simulink model "VB_RIFKF_GNSS_INS25"  (R2023a)
settings: Solver=FixedStepAuto  StartTime=0  StopTime=500  FixedStep=0.01  RelTol=1e-3
InitFcn:
  | resilient_initNavigation1216;
  | init_param;
undefined symbols (not defined in the file or in its folder): dt, g0, gam0_rad, ISUS_flag, magnitude, p, P0, P0_RIEKF, param, pd0, pe0, phi0_rad, pn0, psi, psi0_rad, state_dim, vd0, ve0, vn0
libraries: simulink_extras x68, dspstat3 x54, sharedtransform x47, simulink x43, matrix_library x9, sharedTrackingLibrary x5, dspfactors x4, aerolibconvert2 x3, aerolibtransform2 x3
(part 4 of 22)

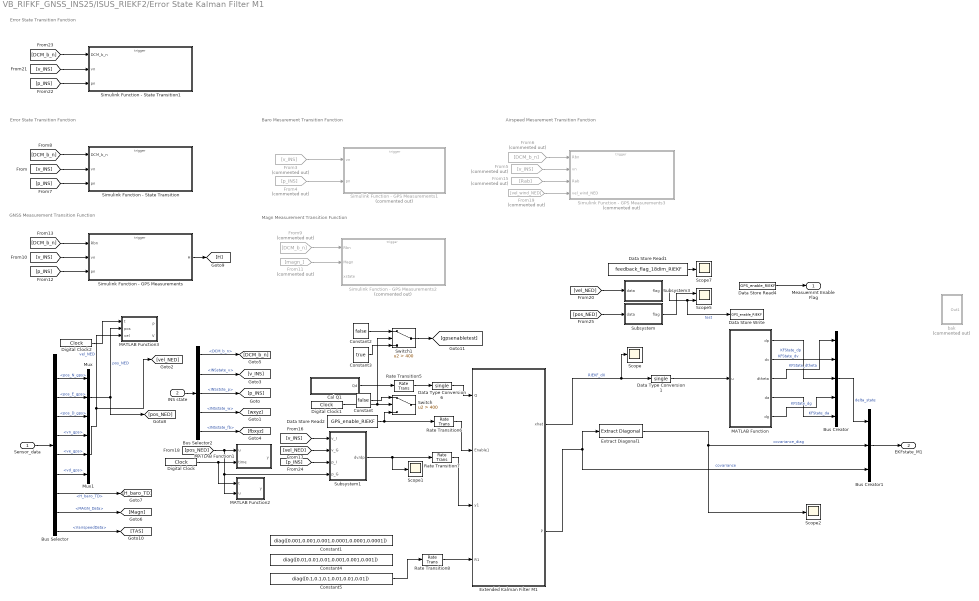
== system VB_RIFKF_GNSS_INS25/ISUS_RIEKF2/Error State Kalman Filter M1 ==
  note: Error State Transition Function
  note: GNSS Measurement Transition Function
  note: Baro Mesurement Transition Function
  note: Magn Measurement Transition Function
  note: Airspeed Mesurement Transition Function
  note: Error State Transition Function
  Sensor_data : Inport
  INS state : Inport  Port=2
  Bus Creator : BusCreator  Inputs=5
  Bus Creator1 : BusCreator  Inputs=3
  Bus Selector : BusSelector  OutputSignals=QGC_sensor_reinit,GPS_Data.pos_N_gps,GPS_Data.pos_E_gps,GPS_Data.pos_D_gps,GPS_Data.vn_gps,GPS_Data.ve_gps,GPS_Data.vd_gps,BARO_Data.H_baro_TD,MAGN_Data,VairspeedData
  Bus Selector2 : BusSelector  OutputSignals=RotationData.DCM_b_n,INSstate_v,INSstste_p,INSstate_w,INSstate_fb
  Cal Q1 : Subsystem
  Constant : Constant  Value=false
  Constant1 : Constant  Value=diag([0.001,0.001,0.001,0.0001,0.0001,0.0001])  OutDataTypeStr=single
  Constant2 : Constant  Value=false
  Constant3 : Constant  Value=true
  Constant4 : Constant  Value=diag([0.01,0.01,0.01,0.001,0.001,0.001])  OutDataTypeStr=single
  Constant5 : Constant  Value=diag([0.1,0.1,0.1,0.01,0.01,0.01])  OutDataTypeStr=single
  Data Store Read1 : DataStoreRead  DataStoreName=feedback_flag_18dim_RIEKF  IndexOptions=Index vector (dialog)  Indices=1  OutputSizes=1
  Data Store Read2 : DataStoreRead  DataStoreName=GPS_enable_RIEKF  IndexOptions=Index vector (dialog)  Indices=1  OutputSizes=1
  Data Store Read4 : DataStoreRead  DataStoreName=GPS_enable_RIEKF  IndexOptions=Index vector (dialog)  Indices=1  OutputSizes=1
  Data Store Write : DataStoreWrite  DataStoreName=GPS_enable_RIEKF  IndexOptions=Index vector (dialog)  Indices=1  OutputSizes=1
  Data Type Conversion1 : DataTypeConversion  OutDataTypeStr=single  SaturateOnIntegerOverflow=off  RndMeth=Floor
  Data Type Conversion6 : DataTypeConversion  OutDataTypeStr=single  SaturateOnIntegerOverflow=off  RndMeth=Floor
  Digital Clock : DigitalClock  SampleTime=0.01
  Digital Clock1 : DigitalClock  SampleTime=0.01
  Digital Clock2 : DigitalClock  SampleTime=0.01
  Extended Kalman Filter M1 : Subsystem  mask(Extended Kalman Filter){StateTransitionFcn=stateTransitionFcn_RIEKF, HasStateTransitionJacobianFcn=on, StateTransitionJacobianFcn=stateFcn_RIEKFJacobian, HasAdditiveProcessNoise=Nonadditive, ProcessNoise=1, HasTimeVaryingProcessNoise=on, HasStateTransitionFcnExtraArgument=0, InitialState=zeros(state_dim,1), InitialStateCovariance=P0_RIEKF, MeasurementFcn1=GPSMeasurementFcn_RIEKF, HasMeasurementJacobianFcn1=off, MeasurementJacobianFcn1=, HasMeasurementEnablePort1=on, HasAdditiveMeasurementNoise1=Nonadditive, MeasurementNoise1=1, HasTimeVaryingMeasurementNoise1=on, HasMeasurementFcnExtraArgument1=0, HasMeasurementWrapping1=off, MeasurementFcn2=BaroMeasurementFcn_RIEKF, HasMeasurementJacobianFcn2=off, MeasurementJacobianFcn2=, HasMeasurementEnablePort2=on, HasAdditiveMeasurementNoise2=Nonadditive, MeasurementNoise2=1, HasTimeVaryingMeasurementNoise2=on, HasMeasurementFcnExtraArgument2=0, HasMeasurementWrapping2=off, MeasurementFcn3=MagnMeasurementFcn_RIEKF, HasMeasurementJacobianFcn3=off, MeasurementJacobianFcn3=, HasMeasurementEnablePort3=on, HasAdditiveMeasurementNoise3=Nonadditive, MeasurementNoise3=1, HasTimeVaryingMeasurementNoise3=on, HasMeasurementFcnExtraArgument3=0, HasMeasurementWrapping3=off, MeasurementFcn4=AirspeedMeasurementFcn_RIEKF, HasMeasurementJacobianFcn4=off, MeasurementJacobianFcn4=, HasMeasurementEnablePort4=on, HasAdditiveMeasurementNoise4=Nonadditive, MeasurementNoise4=1, HasTimeVaryingMeasurementNoise4=on, HasMeasurementFcnExtraArgument4=0, HasMeasurementWrapping4=off, MeasurementFcn5=myMeasurementFcn, HasMeasurementJacobianFcn5=off, MeasurementJacobianFcn5=, HasMeasurementEnablePort5=off, HasAdditiveMeasurementNoise5=Additive, MeasurementNoise5=1, HasTimeVaryingMeasurementNoise5=off, HasMeasurementFcnExtraArgument5=0, HasMeasurementWrapping5=off, EnableMultirate=off, StateTransitionFcnSampleTime=0.01, MeasurementFcn1SampleTime=0.2, MeasurementFcn2SampleTime=0.01, MeasurementFcn3SampleTime=0.01, MeasurementFcn4SampleTime=0.2, MeasurementFcn5SampleTime=1, UseCurrentEstimator=on, OutputStateCovariance=on, DataType=single, SampleTime=0.01, NumberOfMeasurements=1}
      mask prompts: HasStateTransitionJacobianFcn "shared_tracking:blocks:maskPromptEKFJacobian"; HasTimeVaryingProcessNoise "shared_tracking:blocks:maskPromptEKFUKFTimeVarying"; HasMeasurementJacobianFcn1 "shared_tracking:blocks:maskPromptEKFJacobian"; HasMeasurementEnablePort1 "shared_tracking:blocks:maskPromptEnablePort"; HasTimeVaryingMeasurementNoise1 "shared_tracking:blocks:maskPromptEKFUKFTimeVarying"; HasMeasurementWrapping1 "shared_tracking:blocks:maskPromptEKFUKFMeasurementWrapping"; HasMeasurementJacobianFcn2 "shared_tracking:blocks:maskPromptEKFJacobian"; HasMeasurementEnablePort2 "shared_tracking:blocks:maskPromptEnablePort"; HasTimeVaryingMeasurementNoise2 "shared_tracking:blocks:maskPromptEKFUKFTimeVarying"; HasMeasurementWrapping2 "shared_tracking:blocks:maskPromptEKFUKFMeasurementWrapping"; HasMeasurementJacobianFcn3 "shared_tracking:blocks:maskPromptEKFJacobian"; HasMeasurementEnablePort3 "shared_tracking:blocks:maskPromptEnablePort"; HasTimeVaryingMeasurementNoise3 "shared_tracking:blocks:maskPromptEKFUKFTimeVarying"; HasMeasurementWrapping3 "shared_tracking:blocks:maskPromptEKFUKFMeasurementWrapping"; HasMeasurementJacobianFcn4 "shared_tracking:blocks:maskPromptEKFJacobian"; HasMeasurementEnablePort4 "shared_tracking:blocks:maskPromptEnablePort"; HasTimeVaryingMeasurementNoise4 "shared_tracking:blocks:maskPromptEKFUKFTimeVarying"; HasMeasurementWrapping4 "shared_tracking:blocks:maskPromptEKFUKFMeasurementWrapping"; HasMeasurementJacobianFcn5 "shared_tracking:blocks:maskPromptEKFJacobian"; HasMeasurementEnablePort5 "shared_tracking:blocks:maskPromptEnablePort"; HasTimeVaryingMeasurementNoise5 "shared_tracking:blocks:maskPromptEKFUKFTimeVarying"; HasMeasurementWrapping5 "shared_tracking:blocks:maskPromptEKFUKFMeasurementWrapping"; EnableMultirate "shared_tracking:blocks:maskPromptEnableMultirate"; StateTransitionFcnSampleTime "shared_tracking:blocks:maskPromptStateTransition"; MeasurementFcn1SampleTime "shared_tracking:blocks:maskPromptMeasurement1"; MeasurementFcn2SampleTime "shared_tracking:blocks:maskPromptMeasurement2"; MeasurementFcn3SampleTime "shared_tracking:blocks:maskPromptMeasurement3"; MeasurementFcn4SampleTime "shared_tracking:blocks:maskPromptMeasurement4"; MeasurementFcn5SampleTime "shared_tracking:blocks:maskPromptMeasurement5"; UseCurrentEstimator "shared_tracking:blocks:maskPromptUseCurrentEstimator"; OutputStateCovariance "shared_tracking:blocks:maskPromptOutputStateCovariance"; DataType "shared_tracking:blocks:maskPromptDataType"; SampleTime "shared_tracking:blocks:maskPromptSampleTime"
      mask help: shared_tracking:blocks:maskPromptEKFDescription
      mask init:
      | matlabshared.tracking.internal.blocks.maskInitializationScriptEKF
      mask Help: eval('matlabshared.tracking.internal.blocks.controlIdentLaunchDocPage(''EKF'')')
      mask Callback HasStateTransitionJacobianFcn: matlabshared.tracking.internal.blocks.dialogCallbacksEKFUKFPF(gcbh(),'checkBoxHasJacobianFcn','StateTransition');
      mask TypeOptions HasAdditiveProcessNoise: shared_tracking:blocks:maskPromptEKFUKFAdditiveNoise | shared_tracking:blocks:maskPromptEKFUKFNonAdditiveNoise
      mask Callback HasTimeVaryingProcessNoise: matlabshared.tracking.internal.blocks.dialogCallbacksEKFUKFPF(gcbh,'checkboxIsCovarianceTimeVarying','HasTimeVaryingProcessNoise','ProcessNoise')
      mask Callback HasMeasurementJacobianFcn1: matlabshared.tracking.internal.blocks.dialogCallbacksEKFUKFPF(gcbh(),'checkBoxHasJacobianFcn','Measurement','1');
      mask TypeOptions HasAdditiveMeasurementNoise1: shared_tracking:blocks:maskPromptEKFUKFAdditiveNoise | shared_tracking:blocks:maskPromptEKFUKFNonAdditiveNoise
      mask Callback HasTimeVaryingMeasurementNoise1: matlabshared.tracking.internal.blocks.dialogCallbacksEKFUKFPF(gcbh,'checkboxIsCovarianceTimeVarying','HasTimeVaryingMeasurementNoise1','MeasurementNoise1')
      mask Callback HasMeasurementJacobianFcn2: matlabshared.tracking.internal.blocks.dialogCallbacksEKFUKFPF(gcbh(),'checkBoxHasJacobianFcn','Measurement','2');
      mask TypeOptions HasAdditiveMeasurementNoise2: shared_tracking:blocks:maskPromptEKFUKFAdditiveNoise | shared_tracking:blocks:maskPromptEKFUKFNonAdditiveNoise
      mask Callback HasTimeVaryingMeasurementNoise2: matlabshared.tracking.internal.blocks.dialogCallbacksEKFUKFPF(gcbh,'checkboxIsCovarianceTimeVarying','HasTimeVaryingMeasurementNoise2','MeasurementNoise2')
      mask Callback HasMeasurementJacobianFcn3: matlabshared.tracking.internal.blocks.dialogCallbacksEKFUKFPF(gcbh(),'checkBoxHasJacobianFcn','Measurement','3');
      mask TypeOptions HasAdditiveMeasurementNoise3: shared_tracking:blocks:maskPromptEKFUKFAdditiveNoise | shared_tracking:blocks:maskPromptEKFUKFNonAdditiveNoise
      mask Callback HasTimeVaryingMeasurementNoise3: matlabshared.tracking.internal.blocks.dialogCallbacksEKFUKFPF(gcbh,'checkboxIsCovarianceTimeVarying','HasTimeVaryingMeasurementNoise3','MeasurementNoise3')
      mask Callback HasMeasurementJacobianFcn4: matlabshared.tracking.internal.blocks.dialogCallbacksEKFUKFPF(gcbh(),'checkBoxHasJacobianFcn','Measurement','4');
      mask TypeOptions HasAdditiveMeasurementNoise4: shared_tracking:blocks:maskPromptEKFUKFAdditiveNoise | shared_tracking:blocks:maskPromptEKFUKFNonAdditiveNoise
      mask Callback HasTimeVaryingMeasurementNoise4: matlabshared.tracking.internal.blocks.dialogCallbacksEKFUKFPF(gcbh,'checkboxIsCovarianceTimeVarying','HasTimeVaryingMeasurementNoise4','MeasurementNoise4')
      mask Callback HasMeasurementJacobianFcn5: matlabshared.tracking.internal.blocks.dialogCallbacksEKFUKFPF(gcbh(),'checkBoxHasJacobianFcn','Measurement','5');
      mask TypeOptions HasAdditiveMeasurementNoise5: shared_tracking:blocks:maskPromptEKFUKFAdditiveNoise | shared_tracking:blocks:maskPromptEKFUKFNonAdditiveNoise
      mask Callback HasTimeVaryingMeasurementNoise5: matlabshared.tracking.internal.blocks.dialogCallbacksEKFUKFPF(gcbh,'checkboxIsCovarianceTimeVarying','HasTimeVaryingMeasurementNoise5','MeasurementNoise5')
      mask Callback EnableMultirate: matlabshared.tracking.internal.blocks.dialogCallbacksEKFUKFPF(gcbh,'checkBoxHasMultirate')
      mask TypeOptions DataType: shared_tracking:blocks:maskPromptDouble | shared_tracking:blocks:maskPromptSingle
      mask Callback NumberOfMeasurements: matlabshared.tracking.internal.blocks.dialogCallbacksEKFUKFPF(gcbh,'editboxNumberOfMeasurements','MeasurementFcn');
      mask DialogControl DescGroupVar Prompt: shared_tracking:blocks:maskPromptEKFTitle
      mask DialogControl TabSystemModel Prompt: shared_tracking:blocks:maskPromptSystemModel
      mask DialogControl GroupStateTransition Prompt: shared_tracking:blocks:maskPromptStateTransition
      mask DialogControl StateTransitionFunctionText Prompt: shared_tracking:blocks:maskPromptFunction
      mask DialogControl HasStateTransitionJacobianFcn Prompt: Jacobian
      mask DialogControl ProcessNoiseText Prompt: shared_tracking:blocks:maskPromptEKFUKFProcessNoise
      mask DialogControl ProcessNoiseCovarianceText Prompt: shared_tracking:blocks:maskPromptCovariance
      mask DialogControl HasTimeVaryingProcessNoise Prompt: Time-varying
      mask DialogControl InitializationContainer Prompt: shared_tracking:blocks:maskPromptInitialization
      mask DialogControl InitialStateText Prompt: shared_tracking:blocks:maskPromptEKFUKFInitialState
      mask DialogControl InitialCovarianceText Prompt: shared_tracking:blocks:maskPromptEKFUKFInitialCovariance
      mask DialogControl GroupMeasurement1 Prompt: shared_tracking:blocks:maskPromptMeasurement1
      mask DialogControl MeasurementFunction1Text Prompt: shared_tracking:blocks:maskPromptFunction
      mask DialogControl HasMeasurementJacobianFcn1 Prompt: Jacobian
      mask DialogControl HasMeasurementEnablePort1 Prompt: Add Enable port
      mask DialogControl MeasurementNoiseText1 Prompt: shared_tracking:blocks:maskPromptEKFUKFMeasurementNoise
      mask DialogControl MeasurementNoiseCovarianceText1 Prompt: shared_tracking:blocks:maskPromptCovariance
      mask DialogControl HasTimeVaryingMeasurementNoise1 Prompt: Time-varying
      mask DialogControl HasMeasurementWrapping1 Prompt: Has measurement wrapping
      mask DialogControl GroupMeasurement2 Prompt: shared_tracking:blocks:maskPromptMeasurement2
      mask DialogControl MeasurementFunction2Text Prompt: shared_tracking:blocks:maskPromptFunction
      mask DialogControl HasMeasurementJacobianFcn2 Prompt: Jacobian
      mask DialogControl HasMeasurementEnablePort2 Prompt: Add Enable port
      mask DialogControl MeasurementNoiseText2 Prompt: shared_tracking:blocks:maskPromptEKFUKFMeasurementNoise
      mask DialogControl MeasurementNoiseCovarianceText2 Prompt: shared_tracking:blocks:maskPromptCovariance
      mask DialogControl HasTimeVaryingMeasurementNoise2 Prompt: Time-varying
      mask DialogControl HasMeasurementWrapping2 Prompt: Has measurement wrapping
      mask DialogControl GroupMeasurement3 Prompt: shared_tracking:blocks:maskPromptMeasurement3
      mask DialogControl MeasurementFunction3Text Prompt: shared_tracking:blocks:maskPromptFunction
      mask DialogControl HasMeasurementJacobianFcn3 Prompt: Jacobian
      mask DialogControl HasMeasurementEnablePort3 Prompt: Add Enable port
      mask DialogControl MeasurementNoiseText3 Prompt: shared_tracking:blocks:maskPromptEKFUKFMeasurementNoise
      mask DialogControl MeasurementNoiseCovarianceText3 Prompt: shared_tracking:blocks:maskPromptCovariance
      mask DialogControl HasTimeVaryingMeasurementNoise3 Prompt: Time-varying
      mask DialogControl HasMeasurementWrapping3 Prompt: Has measurement wrapping
      mask DialogControl GroupMeasurement4 Prompt: shared_tracking:blocks:maskPromptMeasurement4
      mask DialogControl MeasurementFunction4Text Prompt: shared_tracking:blocks:maskPromptFunction
      mask DialogControl HasMeasurementJacobianFcn4 Prompt: Jacobian
      mask DialogControl HasMeasurementEnablePort4 Prompt: Add Enable port
      mask DialogControl MeasurementNoiseText4 Prompt: shared_tracking:blocks:maskPromptEKFUKFMeasurementNoise
      mask DialogControl MeasurementNoiseCovarianceText4 Prompt: shared_tracking:blocks:maskPromptCovariance
      mask DialogControl HasTimeVaryingMeasurementNoise4 Prompt: Time-varying
      mask DialogControl HasMeasurementWrapping4 Prompt: Has measurement wrapping
      mask DialogControl GroupMeasurement5 Prompt: shared_tracking:blocks:maskPromptMeasurement5
      mask DialogControl MeasurementFunction5Text Prompt: shared_tracking:blocks:maskPromptFunction
      mask DialogControl HasMeasurementJacobianFcn5 Prompt: Jacobian
      mask DialogControl HasMeasurementEnablePort5 Prompt: Add Enable port
      mask DialogControl MeasurementNoiseText5 Prompt: shared_tracking:blocks:maskPromptEKFUKFMeasurementNoise
      mask DialogControl MeasurementNoiseCovarianceText5 Prompt: shared_tracking:blocks:maskPromptCovariance
      mask DialogControl HasTimeVaryingMeasurementNoise5 Prompt: Time-varying
      mask DialogControl HasMeasurementWrapping5 Prompt: Has measurement wrapping
      mask DialogControl AddMeasurement Prompt: shared_tracking:blocks:maskPromptAddMeasurement
      mask DialogControl AddMeasurement Callback: matlabshared.tracking.internal.blocks.dialogCallbacksEKFUKFPF(gcbh,'buttonAddMeasurement','MeasurementFcn');
      mask DialogControl RemoveMeasurement Prompt: shared_tracking:blocks:maskPromptRemoveMeasurement
      mask DialogControl RemoveMeasurement Callback: matlabshared.tracking.internal.blocks.dialogCallbacksEKFUKFPF(gcbh,'buttonRemoveMeasurement','MeasurementFcn');
      mask DialogControl TabMultirate Prompt: shared_tracking:blocks:maskPromptEKFUKFMultirate
      mask DialogControl GroupMultirate Prompt: shared_tracking:blocks:maskPromptEKFUKFMultirate
      mask DialogControl EnableMultirate Prompt: Enable multirate operation
      mask DialogControl GroupMultirateSampleTimes Prompt: shared_tracking:blocks:maskPromptSampleTimeNoInheritance
      mask DialogControl StateTransitionFcnSampleTime Prompt: State Transition
      mask DialogControl MeasurementFcn1SampleTime Prompt: Measurement 1
      mask DialogControl MeasurementFcn2SampleTime Prompt: Measurement 2
      mask DialogControl MeasurementFcn3SampleTime Prompt: Measurement 3
      mask DialogControl MeasurementFcn4SampleTime Prompt: Measurement 4
      mask DialogControl MeasurementFcn5SampleTime Prompt: Measurement 5
      mask DialogControl ContainerSettings Prompt: shared_tracking:blocks:maskPromptEKFUKFSettings
      mask DialogControl UseCurrentEstimator Prompt: Use the current measurements to improve state estimates
      mask DialogControl OutputStateCovariance Prompt: Output state estimation error covariance
      mask DialogControl DataType Prompt: Data type:
      mask DialogControl SampleTime Prompt: Sample time:
  Extract Diagonal1 : matrix_library/Extract Diagonal
  From11 : From  Commented=on  GotoTag=magn_
  From15 : From  Commented=on  GotoTag=Rab
  From19 : From  Commented=on  GotoTag=vel_wind_NED
  From3 : From  Commented=on  GotoTag=v_INS
  From4 : From  Commented=on  GotoTag=p_INS
  From5 : From  Commented=on  GotoTag=v_INS
  From6 : From  Commented=on  GotoTag=DCM_b_n
  From9 : From  Commented=on  GotoTag=DCM_b_n
  MATLAB Function : MATLAB Function  TreatAsAtomicUnit=on
  MATLAB Function1 : MATLAB Function  TreatAsAtomicUnit=on
  MATLAB Function2 : MATLAB Function  TreatAsAtomicUnit=on
  MATLAB Function3 : MATLAB Function  TreatAsAtomicUnit=on
  Mux : Mux  Inputs=3
  Mux1 : Mux  Inputs=3
  Rate Transition{5..8} (4 alike) : RateTransition  OutPortSampleTime=dt
  Scope{,1..2,7} (4 alike) : Scope
  Scope5 : Scope  NumInputPorts=2
  Simulink Function - GPS Measurements : Subsystem  TreatAsAtomicUnit=on
  Simulink Function - GPS Measurements1 : Subsystem  Commented=on  TreatAsAtomicUnit=on
  Simulink Function - GPS Measurements2 : Subsystem  Commented=on  TreatAsAtomicUnit=on
  Simulink Function - GPS Measurements3 : Subsystem  Commented=on  TreatAsAtomicUnit=on
  Simulink Function - State Transition : Subsystem  TreatAsAtomicUnit=on
  Simulink Function - State Transition1 : Subsystem  TreatAsAtomicUnit=on
  Subsystem : Subsystem
  Subsystem1 : Subsystem
  Subsystem3 : Subsystem
  Switch : Switch  Criteria=u2 > Threshold  Threshold=400  SaturateOnIntegerOverflow=off  InputSameDT=off
  Switch1 : Switch  Criteria=u2 > Threshold  Threshold=400  SaturateOnIntegerOverflow=off  InputSameDT=off
  bak : Subsystem  Commented=on
  Measuemrnt Enable Flag : Outport
  EKFstate_M1 : Outport  Port=2
  wires:
  Data Store Read2/1 -> Rate Transition6/1, Switch/3
  Bus Creator/1 -> Bus Creator1/1  "delta_state"
  MATLAB Function/5(dg) -> Bus Creator/4  "KFState_dg"
  MATLAB Function/2(dv) -> Bus Creator/2  "KFState_dv"
  MATLAB Function/4(da) -> Bus Creator/5  "KFState_da"
  Bus Selector2/3 -> [p_INS]  "<INSstste_p>"
  Bus Selector2/1 -> [DCM_b_n]  "<DCM_b_n>"
  Bus Selector2/5 -> [fbxyz]  "<INSstate_fb>"
  Bus Selector2/4 -> [wxyz]  "<INSstate_w>"
  INS state/1 -> Bus Selector2/1
  Bus Selector/4 -> Mux/3  "<pos_D_gps>"
  Bus Selector/2 -> Mux/1  "<pos_N_gps>"
  Bus Selector/3 -> Mux/2  "<pos_E_gps>"
  Bus Selector/7 -> Mux1/3  "<vd_gps>"
  Bus Selector/5 -> Mux1/1  "<vn_gps>"
  Mux1/1 -> [vel_NED], MATLAB Function3/3(vel)  "vel_NED"
  Sensor_data/1 -> Bus Selector/1
  Bus Selector/6 -> Mux1/2  "<ve_gps>"
  Data Store Read1/1 -> Scope7/1
  [pos_NED] -> Subsystem/1(data)
  Subsystem/1(flag) -> Scope5/1
  Extended Kalman Filter M1/1(xhat) -> Scope/1, Data Type Conversion1/1  "RIEKF_dX"
  MATLAB Function/1(dp) -> Bus Creator/3  "KFState_dp"
  MATLAB Function/3(dtheta) -> Bus Creator/1  "KFState_dtheta"
  [DCM_b_n] -> Simulink Function - State Transition/1(DCM_b_n)
  Extended Kalman Filter M1/2(P) -> Bus Creator1/3, Extract Diagonal1/1  "covariance"
  Rate Transition6/1 -> Extended Kalman Filter M1/2(Enable1)
  Cal Q1/1(Qd) -> Rate Transition5/1
  Rate Transition5/1 -> Data Type Conversion6/1
  Data Type Conversion6/1 -> Extended Kalman Filter M1/1(Q)
  Bus Selector2/2 -> [v_INS]  "<INSstate_v>"
  Mux/1 -> MATLAB Function3/2(pos), [pos_NED]  "pos_NED"
  Data Store Read4/1 -> Measuemrnt Enable Flag/1
  [v_INS] -> Simulink Function - State Transition/2(vn)
  [p_INS] -> Simulink Function - State Transition/3(pn)
  Subsystem1/1(dv/dp) -> Rate Transition7/1, Scope1/1
  [v_INS] -> Subsystem1/1(v_I)
  [vel_NED] -> Subsystem1/2(v_G)
  [DCM_b_n] -> Simulink Function - GPS Measurements/1(Rbn)
  [v_INS] -> Simulink Function - GPS Measurements/2(vn)
  [p_INS] -> Simulink Function - GPS Measurements/3(pn)
  Bus Selector/8 -> [H_baro_TD]  "<H_baro_TD>"
  From4/1 -> Simulink Function - GPS Measurements1/2(pn)
  From3/1 -> Simulink Function - GPS Measurements1/1(vn)
  Bus Selector/9 -> [Magn]  "<MAGN_Data>"
  From11/1 -> Simulink Function - GPS Measurements2/2(Magn)
  From9/1 -> Simulink Function - GPS Measurements2/1(Rbn)
  From6/1 -> Simulink Function - GPS Measurements3/1(Rbn)
  From5/1 -> Simulink Function - GPS Measurements3/2(vn)
  Data Type Conversion1/1 -> MATLAB Function/1(u)
  Bus Selector/10 -> [TAS]  "<VairspeedData>"
  From15/1 -> Simulink Function - GPS Measurements3/3(Rab)
  From19/1 -> Simulink Function - GPS Measurements3/4(vel_wind_NED)
  Bus Creator1/1 -> EKFstate_M1/1
  Extract Diagonal1/1 -> Scope2/1, Bus Creator1/2  "covariance_diag"
  [vel_NED] -> Subsystem3/1(data)
  Subsystem3/1(flag) -> Data Store Write/1, Scope5/2  "test"
  [p_INS] -> Simulink Function - State Transition1/3(pn)
  [v_INS] -> Simulink Function - State Transition1/2(vn)
  [DCM_b_n] -> Simulink Function - State Transition1/1(DCM_b_n)
  Rate Transition7/1 -> Extended Kalman Filter M1/3(y1)
  Rate Transition8/1 -> Extended Kalman Filter M1/4(R1)
  Constant5/1 -> Rate Transition8/1
  Simulink Function - GPS Measurements/1(H) -> [H]
  [p_INS] -> Subsystem1/3(p_I)
  Digital Clock/1 -> MATLAB Function2/1(t), MATLAB Function1/2(time)
  [pos_NED] -> MATLAB Function2/2(u), Subsystem1/4(p_G), MATLAB Function1/1(u)
  Digital Clock1/1 -> Switch1/2, Switch/2
  Constant/1 -> Switch/1
  Constant2/1 -> Switch1/1
  Constant3/1 -> Switch1/3
  Switch1/1 -> [gpsenabletest]
  Digital Clock2/1 -> MATLAB Function3/1(t)

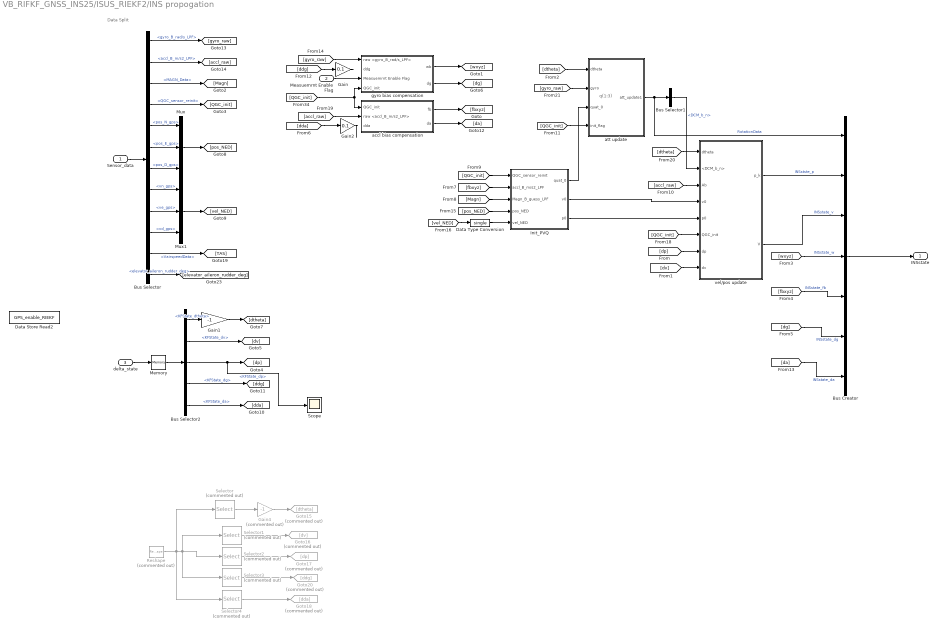
== system VB_RIFKF_GNSS_INS25/ISUS_RIEKF2/INS propogation ==
  note: Data Split
  note: q(1:3)
  Sensor_data : Inport
  Measuemrnt Enable Flag : Inport  Port=2
  delta_state : Inport  Port=3
  Bus Creator : BusCreator  Inputs=7
  Bus Selector : BusSelector  OutputSignals=IMU_Data.gyro_B_rad/s_LPF,IMU_Data.accl_B_m/s2_LPF,MAGN_Data,QGC_sensor_reinit,GPS_Data.pos_N_gps,GPS_Data.pos_E_gps,GPS_Data.pos_D_gps,GPS_Data.vn_gps,GPS_Data.ve_gps,GPS_Data.vd_gps,VairspeedData,elevator_aileron_rudder_deg
  Bus Selector1 : BusSelector  OutputSignals=DCM_b_n
  Bus Selector2 : BusSelector  OutputSignals=KFState_dtheta,KFState_dv,KFState_dp,KFState_dg,KFState_da
  Data Store Read2 : DataStoreRead  DataStoreName=GPS_enable_RIEKF  IndexOptions=Index vector (dialog)  Indices=1  OutputSizes=1
  Data Type Conversion : DataTypeConversion  OutDataTypeStr=single  SaturateOnIntegerOverflow=off  RndMeth=Floor
  Gain : Gain  Gain=0.1
  Gain1 : Gain  Gain=-1
  Gain2 : Gain  Gain=0.1
  Gain4 : Gain  Commented=on  Gain=-1
  Goto15 : Goto  Commented=on  GotoTag=dtheta
  Goto16 : Goto  Commented=on  GotoTag=dv
  Goto17 : Goto  Commented=on  GotoTag=dp
  Goto18 : Goto  Commented=on  GotoTag=dda
  Goto20 : Goto  Commented=on  GotoTag=ddg
  Init_PVQ : Subsystem
  Memory : Memory
  Mux : Mux  Inputs=3
  Mux1 : Mux  Inputs=3
  Reshape : Reshape  Commented=on
  Scope : Scope
  Selector : Selector  Commented=on  InputPortWidth=15  IndexOptions=Index vector (dialog)  Indices=[1 2 3]  OutputSizes=1
  Selector1 : Selector  Commented=on  InputPortWidth=15  IndexOptions=Index vector (dialog)  Indices=[4 5 6]  OutputSizes=1
  Selector2 : Selector  Commented=on  InputPortWidth=15  IndexOptions=Index vector (dialog)  Indices=[7 8 9]  OutputSizes=1
  Selector3 : Selector  Commented=on  InputPortWidth=15  IndexOptions=Index vector (dialog)  Indices=[10 11 12]  OutputSizes=1
  Selector4 : Selector  Commented=on  InputPortWidth=15  IndexOptions=Index vector (dialog)  Indices=[13 14 15]  OutputSizes=1
  accl bias compensation : Subsystem
  att update : Subsystem
  gyro bias compensation : Subsystem
  vel/pos update : Subsystem
  INSstate : Outport
  wires:
  Bus Selector/2 -> [accl_raw]  "<accl_B_m/s2_LPF>"
  [accl_raw] -> accl bias compensation/2(raw <accl_B_m/s2_LPF>)
  [gyro_raw] -> gyro bias compensation/1(raw <gyro_B_rad/s_LPF>)
  Bus Selector2/4 -> [ddg]  "<KFState_dg>"
  Bus Selector2/5 -> [dda]  "<KFState_da>"
  Bus Selector2/1 -> Gain1/1  "<KFState_dtheta>"
  Bus Selector2/2 -> [dv]  "<KFState_dv>"
  Bus Selector2/3 -> Scope/1, [dp]  "<KFState_dp>"
  [da] -> Bus Creator/7  "INSstate_da"
  [dg] -> Bus Creator/6  "INSstate_dg"
  gyro bias compensation/2(dg) -> [dg]
  gyro bias compensation/1(wb) -> [wxyz]
  Measuemrnt Enable Flag/1 -> gyro bias compensation/3(Measuemrnt Enable Flag)
  accl bias compensation/2(da) -> [da]
  accl bias compensation/1(fb) -> [fbxyz]
  att update/1(att_update1) -> Bus Creator/1, Bus Selector1/1  "RotationData"
  [fbxyz] -> Bus Creator/5  "INSstate_fb"
  [wxyz] -> Bus Creator/4  "INSstate_w"
  vel/pos update/1(p_k) -> Bus Creator/2  "INSstste_p"
  [QGC_init] -> Init_PVQ/1(QGC_sensor_reinit)
  [dv] -> vel/pos update/8(dv)
  vel/pos update/2(V) -> Bus Creator/3  "INSstate_v"
  Bus Selector1/1 -> vel/pos update/2(<DCM_b_n>)  "<DCM_b_n>"
  Bus Selector/1 -> [gyro_raw]  "<gyro_B_rad/s_LPF>"
  Bus Selector/4 -> [QGC_init]  "<QGC_sensor_reinit>"
  [Magn] -> Init_PVQ/3(Magn_B_guess_LPF)
  [dp] -> vel/pos update/7(dp)
  Data Type Conversion/1 -> Init_PVQ/5(vel_NED)
  [pos_NED] -> Init_PVQ/4(pos_NED)
  [QGC_init] -> vel/pos update/6(QGC_init)
  Bus Selector/9 -> Mux1/2  "<ve_gps>"
  Init_PVQ/3(p0) -> vel/pos update/5(p0)
  Init_PVQ/2(v0) -> vel/pos update/4(v0)
  [fbxyz] -> Init_PVQ/2(accl_B_m/s2_LPF)
  Sensor_data/1 -> Bus Selector/1
  Mux1/1 -> [vel_NED]
  Bus Selector/3 -> [Magn]  "<MAGN_Data>"
  Bus Selector/6 -> Mux/2  "<pos_E_gps>"
  [gyro_raw] -> att update/2(gyro)
  Bus Selector/5 -> Mux/1  "<pos_N_gps>"
  Bus Selector/8 -> Mux1/1  "<vn_gps>"
  Bus Selector/7 -> Mux/3  "<pos_D_gps>"
  [vel_NED] -> Data Type Conversion/1
  Bus Selector/10 -> Mux1/3  "<vd_gps>"
  [QGC_init] -> att update/4(init_flag)
  [accl_raw] -> vel/pos update/3(Ab)
  Init_PVQ/1(quat_0) -> att update/3(quat_0)
  Mux/1 -> [pos_NED]
  [dtheta] -> vel/pos update/1(dtheta)
  [QGC_init] -> gyro bias compensation/4(QGC_init), accl bias compensation/1(QGC_init)
  Gain1/1 -> [dtheta]
  Bus Selector/11 -> [TAS]  "<VairspeedData>"
  Bus Creator/1 -> INSstate/1
  Bus Selector/12 -> [elevator_aileron_rudder_deg]  "<elevator_aileron_rudder_deg>"
  [ddg] -> Gain/1
  [dda] -> Gain2/1
  [dtheta] -> att update/1(dtheta)
  Memory/1 -> Bus Selector2/1
  Selector3/1 -> Goto20/1
  Selector4/1 -> Goto18/1
  Reshape/1 -> Selector4/1, Selector/1, Selector3/1, Selector1/1, Selector2/1
  Selector2/1 -> Goto17/1
  Selector1/1 -> Goto16/1
  Selector/1 -> Gain4/1
  Gain4/1 -> Goto15/1
  Gain/1 -> ?
  Gain2/1 -> ?
  delta_state/1 -> Memory/1

== system VB_RIFKF_GNSS_INS25/ISUS_RIEKF3/Bus_Constructor ==
  INSstate : Inport
  Bus Creator : BusCreator  Inputs=1
  Bus Creator1 : BusCreator  Inputs=2
  Bus Creator2 : BusCreator  Inputs=6
  Bus Creator4 : BusCreator  Inputs=1
  Bus Selector : BusSelector  OutputSignals=RotationData.DCM_b_n,INSstate_v,INSstste_p,INSstate_dg,INSstate_da
  Data Store Read : DataStoreRead  DataStoreName=GPS_enable_RIEKF  IndexOptions=Index vector (dialog)  Indices=1  OutputSizes=1
  Data Type Conversion : DataTypeConversion  OutDataTypeStr=single  SaturateOnIntegerOverflow=off  RndMeth=Floor
  Demux : Demux  Outputs=3
  Demux1 : Demux  Outputs=3
  Scope : Scope
  TranslationData : Outport
  RotationData : Outport  Port=2
  INSbiasData : Outport  Port=3
  GNSS enable flag : Outport  Port=4
  wires:
  Data Type Conversion/1 -> GNSS enable flag/1
  Bus Creator4/1 -> Data Type Conversion/1
  Data Store Read/1 -> Bus Creator4/1  "GNSS enable flag"
  Bus Creator1/1 -> INSbiasData/1
  Demux/1 -> Bus Creator2/1  "vn_m/s"
  Bus Selector/2 -> Demux/1  "<INSstate_v>"
  Demux1/3 -> Bus Creator2/6  "pd_m"
  Demux1/1 -> Bus Creator2/4  "pn_m"
  Demux1/2 -> Bus Creator2/5  "pe_m"
  Demux/3 -> Bus Creator2/3  "vd_m/s"
  Bus Creator2/1 -> Scope/1, TranslationData/1
  Demux/2 -> Bus Creator2/2  "ve_m/s"
  INSstate/1 -> Bus Selector/1
  Bus Selector/1 -> Bus Creator/1  "<DCM_b_n>"
  Bus Creator/1 -> RotationData/1
  Bus Selector/3 -> Demux1/1  "<INSstste_p>"
  Bus Selector/4 -> Bus Creator1/1  "<INSstate_dg>"
  Bus Selector/5 -> Bus Creator1/2  "<INSstate_da>"

== system VB_RIFKF_GNSS_INS25/ISUS_RIEKF3/Bus_Constructor2 ==
  TranlationData : Inport
  RotationData : Inport  Port=2
  INSbiasData : Inport  Port=3
  GNSS enable flag : Inport  Port=4
  EKFstate_M1 : Inport  Port=5
  EKFstate_M2 : Inport  Port=6
  EKFstate_M3 : Inport  Port=7
  ISIU : Inport  Port=8
  Bus Creator : BusCreator  Inputs=8
  Bus Creator1 : BusCreator  Inputs=3
  Bus Creator2 : BusCreator  Inputs=3
  Bus Creator3 : BusCreator  Inputs=3
  Bus Selector : BusSelector  OutputSignals=delta_state,covariance_diag,m_innov_z0
  Bus Selector1 : BusSelector  OutputSignals=delta_state,covariance_diag,m_innov_z0
  Bus Selector2 : BusSelector  OutputSignals=delta_state,covariance_diag,m_innov_z0
  Rotation_output : Subsystem
  RI EKFNav_out : Outport
  wires:
  Bus Creator3/1 -> Bus Creator/8  "EKFstate_M3"
  Bus Selector2/3 -> Bus Creator3/3  "<m_innov_z0>"
  Bus Selector2/2 -> Bus Creator3/2  "<covariance_diag>"
  Bus Selector2/1 -> Bus Creator3/1  "<delta_state>"
  Bus Creator2/1 -> Bus Creator/7  "EKFstate_M2"
  Bus Selector1/3 -> Bus Creator2/3  "<m_innov_z0>"
  Bus Selector1/2 -> Bus Creator2/2  "<covariance_diag>"
  Bus Selector1/1 -> Bus Creator2/1  "<delta_state>"
  Bus Creator1/1 -> Bus Creator/6  "EKFstate_M1"
  Bus Selector/3 -> Bus Creator1/3  "<m_innov_z0>"
  Bus Selector/2 -> Bus Creator1/2  "<covariance_diag>"
  Bus Selector/1 -> Bus Creator1/1  "<delta_state>"
  EKFstate_M3/1 -> Bus Selector2/1
  EKFstate_M2/1 -> Bus Selector1/1
  EKFstate_M1/1 -> Bus Selector/1
  ISIU/1 -> Bus Creator/5  "ISIU"
  GNSS enable flag/1 -> Bus Creator/4  "GNSS enable flag"
  RotationData/1 -> Rotation_output/1(RotationData)  "RotationData"
  Bus Creator/1 -> RI EKFNav_out/1
  TranlationData/1 -> Bus Creator/1  "TranlationData"
  Rotation_output/1(psi_theta_phi_rad) -> Bus Creator/2  "RotationData"
  INSbiasData/1 -> Bus Creator/3  "INSbiasData"
